simulink model "scdpneumaticlin"  (Simulink 6.0)
settings: Solver=ode23  StartTime=0.0  StopTime=70  FixedStep=1e-3  MaxStep=1  MinStep=1e-3  RelTol=1e-6
model workspace (MAT data in the model file):
  Ts = 294
  Tc = 294
  Tp = 294
  R = 287
  Ps = 700000
  Pe = 100000
  Vp = 0.000128
  Ws = 0.0045
  Ac = 6.16e-06
  Cs = 0.93
  Cc = 0.909
  Vc = 0.0024
  P0 = 200000
  gam : num (value not decoded)
values from neighbouring files (symbols this model uses):
  R = 2    [magballdat.m]
libraries: scddemolib x4
settings Model: Creator=jglass  LastModifiedBy=jglass
settings SolverCC: ZeroCrossControl=EnableAll
settings DataIOCC: SignalLoggingName=logsOut
settings DebuggingCC: CheckExecutionContextPreStartOutputMsg=on  CheckExecutionContextRuntimeOutputMsg=on
settings SFSimCC: SFSimApplyToAllLibs=on  SFSimBuildMode=Incremental

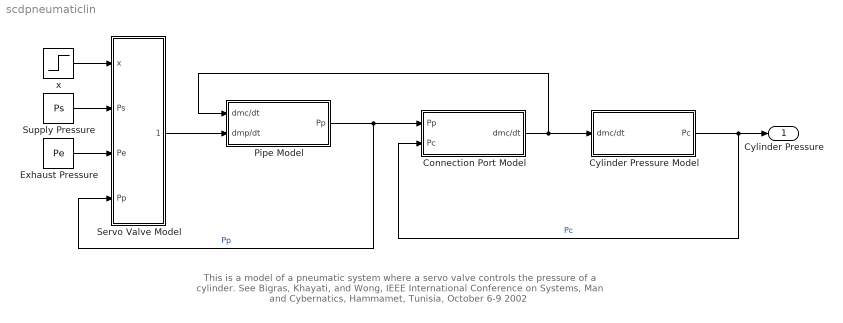
== system scdpneumaticlin ==
  note: This is a model of a pneumatic system where a servo valve controls the pressure of a cylinder.
      | See Bigras, Khayati, and Wong, IEEE International Conference on Systems, Man and Cybernatics, Hammamet, Tunisia, October 6-9 2002
  Connection Port Model : Subsystem  PropExecContextAcrossSSBoundary=on
  Cylinder Pressure Model : Subsystem  PropExecContextAcrossSSBoundary=on
  Exhaust Pressure : Constant  Value=Pe
  Pipe Model : Subsystem  PropExecContextAcrossSSBoundary=on
  Servo Valve Model : Subsystem  PropExecContextAcrossSSBoundary=on
  Supply Pressure : Constant  Value=Ps
  x : Step  After=0.5e-4  SampleTime=0
  Cylinder Pressure : Outport
  wires:
  Supply Pressure/1 -> Servo Valve Model/2(Ps)
  Exhaust Pressure/1 -> Servo Valve Model/3(Pe)
  Pipe Model/1(Pp) -> Servo Valve Model/4(Pp), Connection Port Model/1(Pp)  "Pp"
  Connection Port Model/1(dmc/dt) -> Cylinder Pressure Model/1(dmc/dt), Pipe Model/1(dmc/dt)
  Cylinder Pressure Model/1(Pc) -> Connection Port Model/2(Pc), Cylinder Pressure/1  "Pc"
  Servo Valve Model/1(dmp/dt) -> Pipe Model/2(dmp/dt)
  x/1 -> Servo Valve Model/1(x)

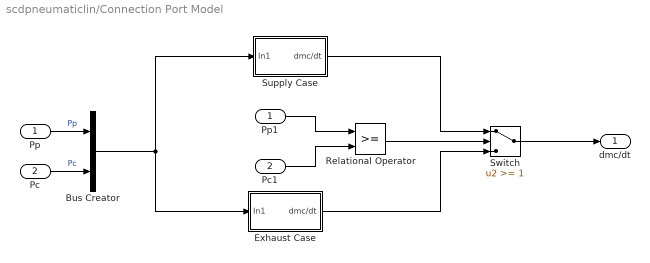
== system scdpneumaticlin/Connection Port Model ==
  Pp : Inport  LatchInput=off
  Pc : Inport  Port=2  LatchInput=off
  Bus Creator : BusCreator  DialogController=Simulink.DDGSource_Bus  Inputs=2
  Exhaust Case : Subsystem  PropExecContextAcrossSSBoundary=on
  Pc1 : InportShadow  Port=2  LatchInput=off
  Pp1 : InportShadow  LatchInput=off
  Relational Operator : RelationalOperator  LogicOutDataTypeMode=Boolean
  Supply Case : Subsystem  PropExecContextAcrossSSBoundary=on
  Switch : Switch  Threshold=1
  dmc/dt : Outport
  wires:
  Pp/1 -> Bus Creator/1  "Pp"
  Pc/1 -> Bus Creator/2  "Pc"
  Bus Creator/1 -> Exhaust Case/1(In1), Supply Case/1(In1)
  Supply Case/1(dmc/dt) -> Switch/1
  Exhaust Case/1(dmc/dt) -> Switch/3
  Switch/1 -> dmc/dt/1
  Relational Operator/1 -> Switch/2
  Pp1/1 -> Relational Operator/1
  Pc1/1 -> Relational Operator/2

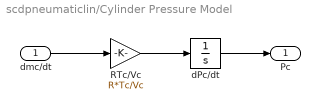
== system scdpneumaticlin/Cylinder Pressure Model ==
  dmc/dt : Inport  LatchInput=off
  RTc/Vc : Gain  Gain=R*Tc/Vc
  dPc/dt : Integrator  InitialCondition=P0  UpperSaturationLimit=0.7e6  LowerSaturationLimit=0
  Pc : Outport
  wires:
  dPc/dt/1 -> Pc/1
  dmc/dt/1 -> RTc/Vc/1
  RTc/Vc/1 -> dPc/dt/1

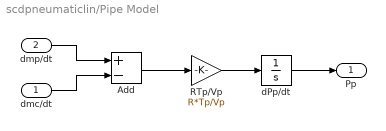
== system scdpneumaticlin/Pipe Model ==
  dmc/dt : Inport  LatchInput=off
  dmp/dt : Inport  Port=2  LatchInput=off
  Add : Sum  Inputs=+-  OutScaling=2^-10
  RTp/Vp : Gain  Gain=R*Tp/Vp
  dPp/dt : Integrator  InitialCondition=P0  UpperSaturationLimit=0.7e6  LowerSaturationLimit=0
  Pp : Outport
  wires:
  RTp/Vp/1 -> dPp/dt/1
  dPp/dt/1 -> Pp/1
  dmp/dt/1 -> Add/1
  dmc/dt/1 -> Add/2
  Add/1 -> RTp/Vp/1

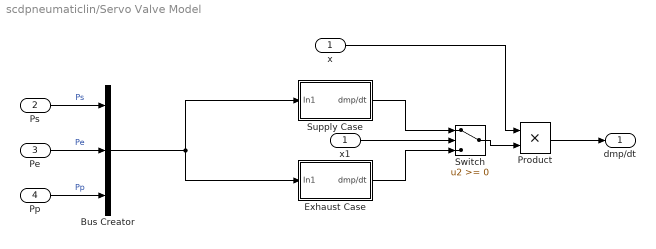
== system scdpneumaticlin/Servo Valve Model ==
  x : Inport  LatchInput=off
  Ps : Inport  Port=2  LatchInput=off
  Pe : Inport  Port=3  LatchInput=off
  Pp : Inport  Port=4  LatchInput=off
  Bus Creator : BusCreator  DialogController=Simulink.DDGSource_Bus  Inputs=3
  Exhaust Case : Subsystem  PropExecContextAcrossSSBoundary=on
  Product : Product  RndMeth=Zero
  Supply Case : Subsystem  PropExecContextAcrossSSBoundary=on
  Switch : Switch
  x1 : InportShadow  LatchInput=off
  dmp/dt : Outport
  wires:
  x/1 -> Product/1
  Ps/1 -> Bus Creator/1  "Ps"
  Pe/1 -> Bus Creator/2  "Pe"
  Pp/1 -> Bus Creator/3  "Pp"
  Bus Creator/1 -> Supply Case/1(In1), Exhaust Case/1(In1)
  Switch/1 -> Product/2
  Product/1 -> dmp/dt/1
  Supply Case/1(dmp/dt) -> Switch/1
  x1/1 -> Switch/2
  Exhaust Case/1(dmp/dt) -> Switch/3

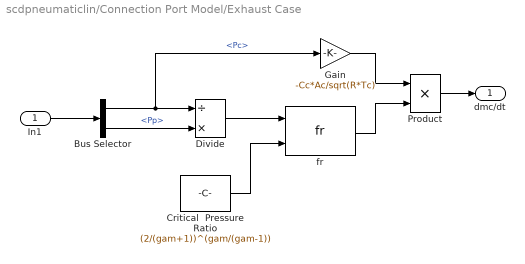
== system scdpneumaticlin/Connection Port Model/Exhaust Case ==
  In1 : Inport  LatchInput=off
  Bus Selector : BusSelector  DialogController=Simulink.DDGSource_Bus  OutputSignals=Pc,Pp
  Critical  Pressure Ratio : Constant  Value=(2/(gam+1))^(gam/(gam-1))
  Divide : Product  Inputs=/*  OutScaling=2^-10
  Gain : Gain  Gain=-Cc*Ac/sqrt(R*Tc)
  Product : Product  Inputs=**  OutScaling=2^-10
  fr : scddemolib/fr
  dmc/dt : Outport
  wires:
  fr/1 -> Product/2
  Critical  Pressure Ratio/1 -> fr/2
  Divide/1 -> fr/1
  Gain/1 -> Product/1
  Product/1 -> dmc/dt/1
  In1/1 -> Bus Selector/1
  Bus Selector/1 -> Gain/1, Divide/1  "<Pc>"
  Bus Selector/2 -> Divide/2  "<Pp>"

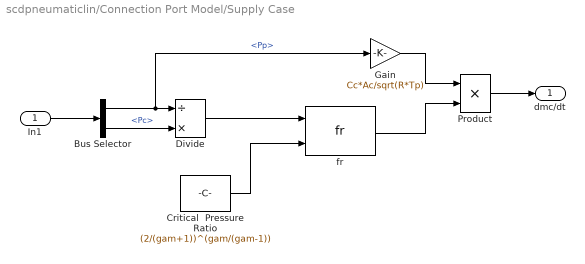
== system scdpneumaticlin/Connection Port Model/Supply Case ==
  In1 : Inport  LatchInput=off
  Bus Selector : BusSelector  DialogController=Simulink.DDGSource_Bus  OutputSignals=Pp,Pc
  Critical  Pressure Ratio : Constant  Value=(2/(gam+1))^(gam/(gam-1))
  Divide : Product  Inputs=/*  OutScaling=2^-10
  Gain : Gain  Gain=Cc*Ac/sqrt(R*Tp)
  Product : Product  Inputs=**  OutScaling=2^-10
  fr : scddemolib/fr
  dmc/dt : Outport
  wires:
  fr/1 -> Product/2
  Critical  Pressure Ratio/1 -> fr/2
  Divide/1 -> fr/1
  Gain/1 -> Product/1
  Product/1 -> dmc/dt/1
  In1/1 -> Bus Selector/1
  Bus Selector/1 -> Divide/1, Gain/1  "<Pp>"
  Bus Selector/2 -> Divide/2  "<Pc>"

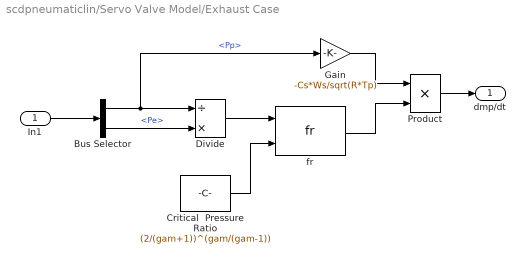
== system scdpneumaticlin/Servo Valve Model/Exhaust Case ==
  In1 : Inport  LatchInput=off
  Bus Selector : BusSelector  DialogController=Simulink.DDGSource_Bus  OutputSignals=Pp,Pe
  Critical  Pressure Ratio : Constant  Value=(2/(gam+1))^(gam/(gam-1))
  Divide : Product  Inputs=/*  OutScaling=2^-10
  Gain : Gain  Gain=-Cs*Ws/sqrt(R*Tp)
  Product : Product  Inputs=**  OutScaling=2^-10
  fr : scddemolib/fr
  dmp/dt : Outport
  wires:
  In1/1 -> Bus Selector/1
  Bus Selector/1 -> Gain/1, Divide/1  "<Pp>"
  Bus Selector/2 -> Divide/2  "<Pe>"
  Product/1 -> dmp/dt/1
  Gain/1 -> Product/1
  Divide/1 -> fr/1
  Critical  Pressure Ratio/1 -> fr/2
  fr/1 -> Product/2

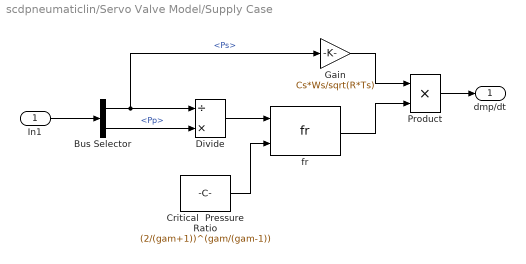
== system scdpneumaticlin/Servo Valve Model/Supply Case ==
  In1 : Inport  LatchInput=off
  Bus Selector : BusSelector  DialogController=Simulink.DDGSource_Bus  OutputSignals=Ps,Pp
  Critical  Pressure Ratio : Constant  Value=(2/(gam+1))^(gam/(gam-1))
  Divide : Product  Inputs=/*  OutScaling=2^-10
  Gain : Gain  Gain=Cs*Ws/sqrt(R*Ts)
  Product : Product  Inputs=**  OutScaling=2^-10
  fr : scddemolib/fr
  dmp/dt : Outport  InitialOutput=10
  wires:
  In1/1 -> Bus Selector/1
  Product/1 -> dmp/dt/1
  Gain/1 -> Product/1
  Divide/1 -> fr/1
  Critical  Pressure Ratio/1 -> fr/2
  fr/1 -> Product/2
  Bus Selector/2 -> Divide/2  "<Pp>"
  Bus Selector/1 -> Divide/1, Gain/1  "<Ps>"
